simulink model "fsk"  (R2018a)
settings: Solver=VariableStepAuto  StartTime=0.0  StopTime=10.0  RelTol=1e-3
libraries: commrandsrc3 x1
settings Model: Creator=hp  LastModifiedBy=hp

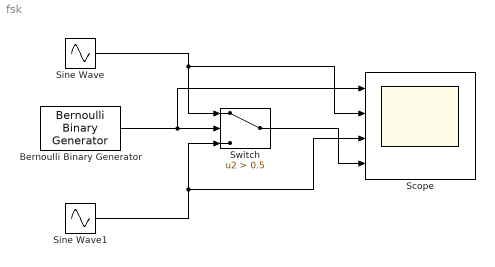
== system fsk ==
  Bernoulli Binary Generator : commrandsrc3/Bernoulli Binary Generator  ProbabilityOfZero=0.5  SeedSource=Auto  Seed=0  SampleTime=1  SamplesPerFrame=1  OutputDataType=double  SimulateUsing=Interpreted execution
  Scope : Scope  NumInputPorts=4
  Sine Wave : Sin  Frequency=100  SampleTime=0.01
  Sine Wave1 : Sin  SampleTime=0.01
  Switch : Switch  Criteria=u2 > Threshold  Threshold=0.5
  wires:
  Bernoulli Binary Generator/1 -> Scope/1, Switch/2
  Sine Wave/1 -> Scope/2, Switch/1
  Sine Wave1/1 -> Scope/3, Switch/3
  Switch/1 -> Scope/4
